simulink model "px4demo_HostSerial_TxRx_total"  (R2016b)
settings: Solver=FixedStepAuto  StartTime=0.0  StopTime=inf  FixedStep=0.005  RelTol=1e-3  EnableMultiTasking=on
undefined symbols (not defined in the file or in its folder): serial
libraries: instrumentlib x3, aerolibanimutils x1
settings Model: Creator=darenlee  LastModifiedBy=E6320
settings DataIOCC: LimitDataPoints=on
settings OptimizationCC: LifeSpan=inf
settings DebuggingCC: ParameterOverflowMsg=none  AllowSymbolicDim=off  SFUnexpectedBacktrackingDiag=warning  SFNoUnconditionalDefaultTransitionDiag=warning  SFExecutionAtInitializationDiag=none
settings ModelReferenceCC: PropagateSignalLabelsOutOfModel=off
settings GRTTargetCC: TargetLangStandard=C89/C90 (ANSI)
settings ConfigComp: CovMetricSettings=dw  CovHtmlReporting=on  CovSaveCumulativeToWorkspaceVar=on  CovSaveSingleToWorkspaceVar=on  CovExternalEMLEnable=off

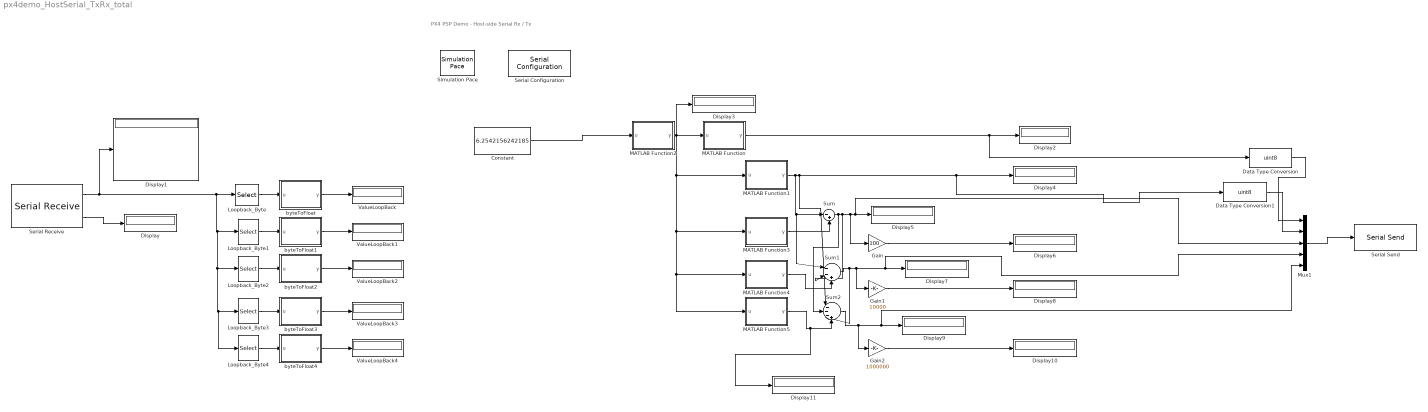
== system px4demo_HostSerial_TxRx_total ==
  note: PX4 PSP Demo - Host-side Serial Rx / Tx
  Constant : Constant  Value=6.2542156242185  SampleTime=0.005
  Data Type Conversion : DataTypeConversion  OutDataTypeStr=uint8
  Data Type Conversion1 : DataTypeConversion  OutDataTypeStr=uint8
  Display{,1..11} (12 alike) : Display
  Gain : Gain  Gain=100
  Gain1 : Gain  Gain=10000
  Gain2 : Gain  Gain=1000000
  Loopback_Byte : Selector  InputPortWidth=8  IndexOptions=Index vector (dialog)  Indices=1:4  OutputSizes=1
  Loopback_Byte1 : Selector  InputPortWidth=8  IndexOptions=Index vector (dialog)  Indices=5:8  OutputSizes=1
  Loopback_Byte2 : Selector  InputPortWidth=20  IndexOptions=Index vector (dialog)  Indices=9:12  OutputSizes=1
  Loopback_Byte3 : Selector  InputPortWidth=20  IndexOptions=Index vector (dialog)  Indices=13:16  OutputSizes=1
  Loopback_Byte4 : Selector  InputPortWidth=20  IndexOptions=Index vector (dialog)  Indices=17:20  OutputSizes=1
  MATLAB Function : MATLAB Function  TreatAsAtomicUnit=on
  MATLAB Function1 : MATLAB Function  TreatAsAtomicUnit=on
  MATLAB Function2 : MATLAB Function  TreatAsAtomicUnit=on
  MATLAB Function3 : MATLAB Function  TreatAsAtomicUnit=on
  MATLAB Function4 : MATLAB Function  TreatAsAtomicUnit=on
  MATLAB Function5 : MATLAB Function  TreatAsAtomicUnit=on
  Mux1 : Mux  Inputs=5
  Serial Configuration : instrumentlib/Serial Configuration  Priority=-200000  ComPortMenu=<Please select a port...>  ComPort=COM7  ObjConstructor=serial('COM7');  BaudRate=57600  DataBits=8  Parity=none  StopBits=1  FlowControl=none  Timeout=10  ByteOrder=LittleEndian
  Serial Receive : instrumentlib/Serial Receive  ComPortMenu=<Please select a port...>  ComPort=COM7  ObjConstructor=serial('COM7');  Terminator=<none>  DataSize="[8  1]"  DataType=uint8  EnableBlockingMode=off  ActionDataUnavailable=Output last received value  CustomValue=0  SampleTime=0.5
  Serial Send : instrumentlib/Serial Send  ComPortMenu=<Please select a port...>  ComPort=COM7  ObjConstructor=serial('COM7');  Terminator=<none>  EnableBlockingMode=off
  Simulation Pace : aerolibanimutils/Simulation Pace  SimulationPace=1  SleepMode=MATLAB Thread  OutputPaceError=off  SampleTime=0.5
  Sum : Sum  Inputs=|-+
  Sum1 : Sum  Inputs=|--+
  Sum2 : Sum  Inputs=|---+
  ValueLoopBack{,1..4} (5 alike) : Display
  byteToFloat : MATLAB Function  TreatAsAtomicUnit=on
  byteToFloat1 : MATLAB Function  TreatAsAtomicUnit=on
  byteToFloat2 : MATLAB Function  TreatAsAtomicUnit=on
  byteToFloat3 : MATLAB Function  TreatAsAtomicUnit=on
  byteToFloat4 : MATLAB Function  TreatAsAtomicUnit=on
  wires:
  Serial Receive/1 -> Loopback_Byte4/1, Loopback_Byte3/1, Loopback_Byte2/1, Loopback_Byte1/1, Loopback_Byte/1, Display1/1
  Loopback_Byte/1 -> byteToFloat/1(u)
  byteToFloat/1(y) -> ValueLoopBack/1
  MATLAB Function/1(y) -> Data Type Conversion/1, Display2/1
  MATLAB Function2/1(y) -> MATLAB Function5/1(u), MATLAB Function4/1(u), MATLAB Function3/1(u), MATLAB Function1/1(u), Display3/1, MATLAB Function/1(u)
  Constant/1 -> MATLAB Function2/1(u)
  MATLAB Function1/1(y) -> Sum1/1, Sum/1, Sum2/1, Data Type Conversion1/1, Display4/1
  Sum/1 -> Sum2/2, Sum1/2, Gain/1, Mux1/3, Display5/1
  MATLAB Function3/1(y) -> Sum/2
  Gain/1 -> Display6/1
  MATLAB Function4/1(y) -> Sum1/3
  Gain1/1 -> Display8/1
  MATLAB Function5/1(y) -> Display11/1, Sum2/4
  Sum2/1 -> Gain2/1, Mux1/5, Display9/1
  Gain2/1 -> Display10/1
  Sum1/1 -> Sum2/3, Gain1/1, Mux1/4, Display7/1
  Loopback_Byte1/1 -> byteToFloat1/1(u)
  byteToFloat1/1(y) -> ValueLoopBack1/1
  Loopback_Byte2/1 -> byteToFloat2/1(u)
  byteToFloat2/1(y) -> ValueLoopBack2/1
  Loopback_Byte3/1 -> byteToFloat3/1(u)
  byteToFloat3/1(y) -> ValueLoopBack3/1
  Loopback_Byte4/1 -> byteToFloat4/1(u)
  byteToFloat4/1(y) -> ValueLoopBack4/1
  Serial Receive/2 -> Display/1
  Mux1/1 -> Serial Send/1
  Data Type Conversion/1 -> Mux1/1
  Data Type Conversion1/1 -> Mux1/2

== matlab function px4demo_HostSerial_TxRx_total/MATLAB Function1 ==
  data: u input; y output
function y = fcn(u)
y = abs(u)
y=floor(y);
end

== matlab function px4demo_HostSerial_TxRx_total/MATLAB Function ==
  data: u input; y output
function y = fcn(u)
if(u<0)
y=99
elseif(u>0)
    y=88
else
    y=0
end

== matlab function px4demo_HostSerial_TxRx_total/MATLAB Function2 ==
  data: u input; y output
function y = fcn(u)
y = floor(u*1000000)/1000000;
end

== matlab function px4demo_HostSerial_TxRx_total/MATLAB Function3 ==
  data: u input; y output
function y = fcn(u)
y = abs(u)
y=floor(y*100)/100;
end

== matlab function px4demo_HostSerial_TxRx_total/MATLAB Function4 ==
  data: u input; y output
function y = fcn(u)
y = abs(u)
y=floor(y*10000)/10000;
end

== matlab function px4demo_HostSerial_TxRx_total/MATLAB Function5 ==
  data: u input; y output
function y = fcn(u)
y = abs(u)
y=floor(y*1000000)/1000000;
end

== matlab function px4demo_HostSerial_TxRx_total/byteToFloat ==
  data: u input; y output
function y = fcn(u)
%#codegen
y = single(0);
y = single(typecast(uint8(u),'single'));
% y = u;

== matlab function px4demo_HostSerial_TxRx_total/byteToFloat1 ==
  data: u input; y output
function y = fcn(u)
%#codegen
y = single(0);
y = single(typecast(uint8(u),'single'));
% y = u;

== matlab function px4demo_HostSerial_TxRx_total/byteToFloat2 ==
  data: u input; y output
function y = fcn(u)
%#codegen
y = single(0);
y = single(typecast(uint8(u),'single'));
% y = u;

== matlab function px4demo_HostSerial_TxRx_total/byteToFloat3 ==
  data: u input; y output
function y = fcn(u)
%#codegen
y = single(0);
y = single(typecast(uint8(u),'single'));
% y = u;

== matlab function px4demo_HostSerial_TxRx_total/byteToFloat4 ==
  data: u input; y output
function y = fcn(u)
%#codegen
y = single(0);
y = single(typecast(uint8(u),'single'));
% y = u;
